simulink model "RL_GHV_open_smc"  (R2023b)
settings: Solver=VariableStepAuto  StartTime=0  StopTime=5  FixedStep=0.01  MaxStep=0.001  RelTol=1e-3
model workspace (MAT data in the model file):
  initPosLLA = [0; 0; 30000]
values from neighbouring files (symbols this model uses):
  Vm_0 = [speed_0; 0; 0]    [init_RL_GHV_open_evn_agent.m]
undefined symbols (not defined in the file or in its folder): e0_0, e1_0, e2_0, e3_0, GHV_cfg, LLA_init, pm_0, Speed_init
libraries: aerolib6dof2 x6, sharedutil x4, aerolibtransform2 x4, sharedtransform x4, simulink_extras x4, shared6dofsys x3, aerolibasang x3, aerolibatmos2 x1, matrix_library x1, aerolibgravity2 x1, rllib x1
settings Model: SimulationMode=accelerator  Creator=Admin  LastModifiedBy=Admin
settings SolverCC: AllowMultiTaskInputOutput=on  ZeroCrossControl=EnableAll  ZeroCrossAlgorithm=Adaptive  AutoInsertRateTranBlk=on
settings DebuggingCC: IgnoredZcDiagnostic=none

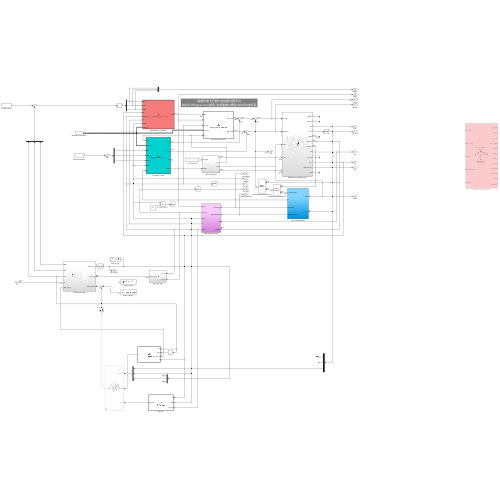
[thumbnail: Simulink's stored preview of the top-level diagram]
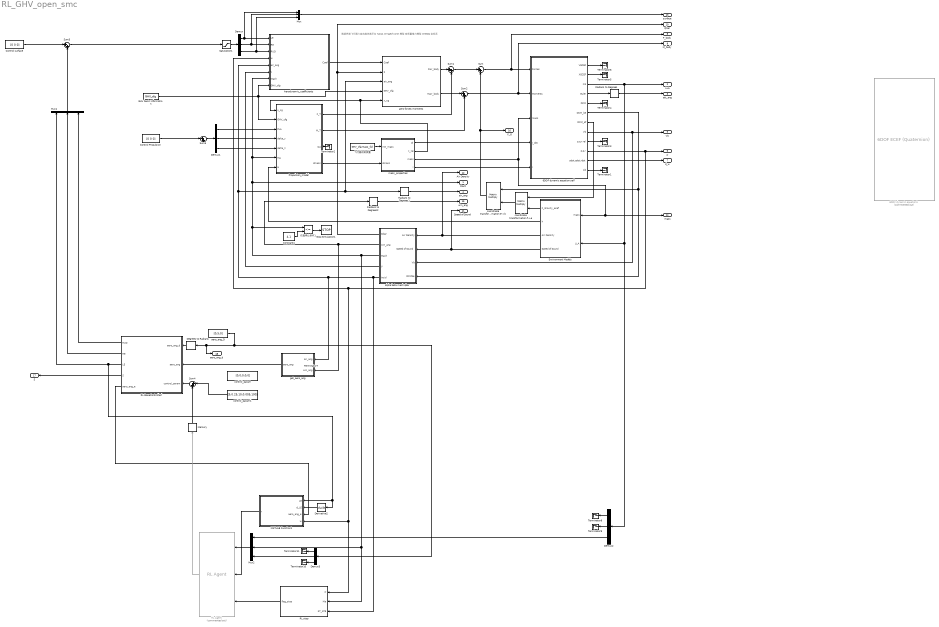
== system RL_GHV_open_smc ==
  note: 高超声速飞行器六自由度仿真平台
      | NASA Winged-cone模型 变质量推力模型 WGS84坐标系
  6DOF dynamic equation self : Subsystem
  6DOF dynamic equation1 : aerolib6dof2/6DOF ECEF (Quaternion)  Commented=on  units=Metric (MKS)  mtype=Custom Variable  xg_0=[0;0;20000]  Vm_0=[1475.347986769521;0;0]  eul_0=[0;0;0]  pm_0=[0;0;0]  mass_0=1.0  mass_e=0.5  mass_f=2.0  inertia=eye(3)  inertia_e=eye(3)  inertia_f=2*eye(3)  vre_flag=off  abi_flag=off  ptype=Custom  R=6378137  F=1/298.257223563  w_E=0  angle_in=Internal  LPM0=0  quat_statename=''  pm_statename=''  Vm_statename=''  posfixedframe_statename=''  posinertial_statename=''  LPM_statename=''  mass_statename=''
      settings: LibrarySourceBlock=|
      | aerolib6dof2/Custom Variable Mass 6DOF
      | ECEF (Quaternion)
  Aerodynamic_coefficients : MATLAB Function  TreatAsAtomicUnit=on
  Constant1 : Constant  Value=4.1
  Control Propulsion : Constant  Value=[0 0 0]
  Control surface : Constant  Value=[0 0 0]
  Degrees to Radians : simulink_extras/Transformations/Degrees to Radians
  Demux{,1..3} (4 alike) : Demux  Outputs=3
  Derivative2 : Derivative
  Environment Models : Subsystem
  GHV basic information : Constant  Value=GHV_cfg  VectorParams1D=off  OutDataTypeStr=Bus: slBus1
  MATLAB Function1 : MATLAB Function  TreatAsAtomicUnit=on
  Memory : Memory
  Mux : Mux  Inputs=3
  Mux1 : Mux  Inputs=3
  Mux2 : Mux  Inputs=3
  Propulsion_model : MATLAB Function  TreatAsAtomicUnit=on
  RL Agent : rllib/RL Agent  Commented=on  Agent=agent1_Trained  ExternalActionAsInput=off  ProvideLastAction=off  ProvideCumRwd=off  TreatAsDirectFeedthrough=on  UseStrictObservationDataTypes=off
  RL BaseControllerl : Subsystem
  RL stop : MATLAB Function  TreatAsAtomicUnit=on
  Radians to Degrees : simulink_extras/Transformations/Radians to Degrees
  Radians to Degrees1 : simulink_extras/Transformations/Radians to Degrees
  Radians to Degrees2 : simulink_extras/Transformations/Radians to Degrees
  Saturation1 : Saturate  UpperLimit=30  LowerLimit=-30
  Stop Simulation1 : Stop
  Sum{,1..5} (6 alike) : Sum  Inputs=|++
  Terminator{1..11} (11 alike) : Terminator
  aero forces moments : MATLAB Function  TreatAsAtomicUnit=on
  aero_ang_D : Constant  Value=[0;5;0]
  alpha beta mach qbar : Subsystem
  control_param : Constant  Value=[0;0;0;0;0]
  control_param1 : Constant  Value=[5;0.25;10;0.005;100]
  coordinate transformation e->b : Product  Multiplication=Matrix(*)
  coordinate transformation f->e : Product  Multiplication=Matrix(*)
  get_aero_ang : Subsystem
  mass_properties : Subsystem
  仿真停止条件1 : RelationalOperator  Operator=<=  OutDataTypeStr=boolean  RndMeth=Simplest  InputSameDT=off
  飞行器初始质量 : Constant  Value=GHV_cfg.mass_full
  Mach : Outport
  LLA : Outport  Port=2
  att_ang : Outport  Port=3
  air_ang : Outport  Port=4
  Vb : Outport  Port=5
  w : Outport  Port=6
  d_w : Outport  Port=7
  F_body : Outport  Port=8
  M_body : Outport  Port=9
  Qbar : Outport  Port=10
  Speed of Sound : Outport  Port=11
  Air Density : Outport  Port=12
  surface : Outport  Port=13
  mass : Outport  Port=14
  win_ang : Outport  Port=15
  F_G : Outport  Port=16
  S : Outport  Port=17
  aero_ang_d : Outport  Port=18
  wires:
  Control surface/1 -> Sum3/1
  coordinate transformation e->b/1 -> F_G/1, Sum/2
  Aerodynamic_coefficients/1(Coef) -> aero forces moments/1(Coef)
  mass_properties/2(x_cg) -> Propulsion_model/1(x_cg), aero forces moments/5(x_cg)
  coordinate transformation f->e/1 -> coordinate transformation e->b/2
  飞行器初始质量/1 -> mass_properties/1(init_mass)
  Radians to Degrees1/1 -> air_ang/1
  Propulsion_model/2(M_T) -> Sum2/2
  6DOF dynamic equation self/1(VECEF) -> Terminator6/1
  6DOF dynamic equation self/9(p,q,r rel) -> Terminator3/1
  mass_properties/3(mass) -> 6DOF dynamic equation self/3(mass), Environment Models/1(mass), mass/1
  Radians to Degrees2/1 -> win_ang/1
  Demux/1 -> Aerodynamic_coefficients/1(LE), Mux/1
  6DOF dynamic equation self/5(DCM) -> Terminator4/1
  Saturation1/1 -> Demux/1
  Demux1/2 -> Propulsion_model/4(delta_y)
  Control Propulsion/1 -> Sum5/1
  Propulsion_model/1(F_T) -> Sum1/2
  6DOF dynamic equation self/3(XG) -> LLA/1, Environment Models/2(LLA), Demux2/1
  Demux/2 -> Aerodynamic_coefficients/2(RE), Mux/2
  alpha beta mach qbar/5(Incid) -> aero forces moments/3(air_ang), Radians to Degrees1/1, Aerodynamic_coefficients/5(air_ang), get_aero_ang/1(air_ang), RL stop/3(air_ang)
  Sum2/1 -> 6DOF dynamic equation self/2(Moments), M_body/1
  Propulsion_model/4(dmass) -> mass_properties/2(dmass)
  Sum1/1 -> Sum/1
  Environment Models/3(Air Density) -> alpha beta mach qbar/1(Air Density), Air Density/1
  Environment Models/2(h) -> Propulsion_model/7(H)
  alpha beta mach qbar/1(Qbar) -> aero forces moments/2(q), Qbar/1
  aero forces moments/1(Fair_body) -> Sum1/1
  Radians to Degrees/1 -> att_ang/1
  6DOF dynamic equation self/6(DCM_be) -> alpha beta mach qbar/4(DCMbe), coordinate transformation e->b/1
  aero forces moments/2(Mair_body) -> Sum2/1
  Demux1/3 -> Propulsion_model/5(delta_z)
  6DOF dynamic equation self/10(p,q,r) -> w/1, RL stop/1(w), MATLAB Function1/4(w), Aerodynamic_coefficients/4(w)
  Mux/1 -> surface/1
  GHV basic information/1 -> Propulsion_model/2(GHV_cfg), aero forces moments/4(GHV_cfg), Aerodynamic_coefficients/8(GHV_cfg)
  Demux/3 -> Aerodynamic_coefficients/3(RUD), Mux/3
  alpha beta mach qbar/2(win_ang) -> Radians to Degrees2/1, get_aero_ang/2(win_ang)
  Sum3/1 -> Saturation1/1
  Propulsion_model/3(Isp) -> Terminator2/1
  Environment Models/1(F_Gravity_ecef) -> coordinate transformation f->e/2
  6DOF dynamic equation self/11(pdot,qdot,rdot) -> d_w/1
  Demux1/1 -> Propulsion_model/3(PLA)
  mass_properties/1(dI) -> 6DOF dynamic equation self/4(I_dot)
  6DOF dynamic equation self/7(DCM_ef) -> coordinate transformation f->e/1
  6DOF dynamic equation self/2(XECEF) -> Terminator5/1
  6DOF dynamic equation self/8(Vb) -> Vb/1, alpha beta mach qbar/3(Vb)
  alpha beta mach qbar/4(V) -> Aerodynamic_coefficients/6(v)
  Environment Models/4(Speed of Sound) -> alpha beta mach qbar/2(Speed of Sound), Speed of Sound/1
  6DOF dynamic equation self/12(Ab) -> Terminator1/1
  6DOF dynamic equation self/4(Euler) -> Radians to Degrees/1
  Sum/1 -> 6DOF dynamic equation self/1(Forces), F_body/1
  mass_properties/4(I) -> 6DOF dynamic equation self/5(I)
  Sum5/1 -> Demux1/1
  alpha beta mach qbar/3(Mach) -> 仿真停止条件1/1, Mach/1, Propulsion_model/6(Ma), Aerodynamic_coefficients/7(Mach), RL stop/2(Ma), Mux2/2
  Mux1/1 -> Sum3/2
  Constant1/1 -> 仿真停止条件1/2
  仿真停止条件1/1 -> Stop Simulation1/1
  get_aero_ang/1(aero_ang) -> RL BaseControllerl/2(aero_ang)
  aero_ang_D/1 -> Demux3/1, aero_ang_d/1, Degrees to Radians/1
  RL BaseControllerl/1(RUD) -> Mux1/3
  RL BaseControllerl/2(RE) -> Mux1/2
  RL BaseControllerl/3(LE) -> MATLAB Function1/1(LE), Derivative2/1, Mux1/1
  RL BaseControllerl/4(S) -> S/1
  Degrees to Radians/1 -> RL BaseControllerl/1(aero_ang_d)
  Sum4/1 -> RL BaseControllerl/3(control_param)
  RL stop/1(flag_stop) -> RL Agent/3
  RL BaseControllerl/5(aero_ang_e) -> MATLAB Function1/3(aero_ang_e)
  MATLAB Function1/1(r) -> RL Agent/2
  Mux2/1 -> RL Agent/1
  Demux2/1 -> Terminator8/1
  Demux2/2 -> Terminator9/1
  Demux2/3 -> Mux2/1
  RL Agent/1 -> Memory/1
  control_param1/1 -> Sum4/1
  Derivative2/1 -> MATLAB Function1/2(d_LE)
  Demux3/2 -> Mux2/3
  Demux3/3 -> Terminator10/1
  Demux3/1 -> Terminator11/1
  Memory/1 -> Sum4/2

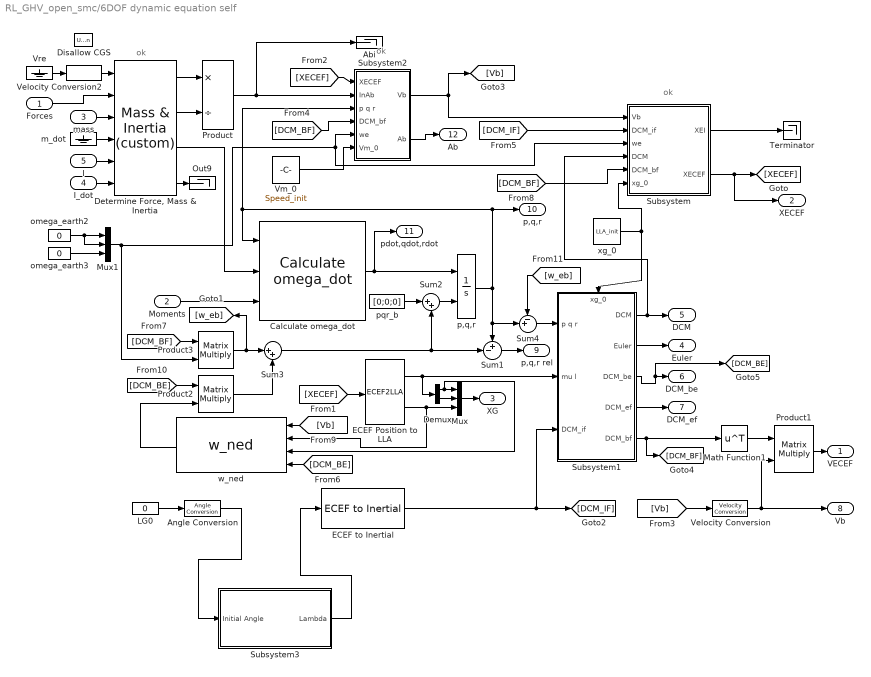
== system RL_GHV_open_smc/6DOF dynamic equation self ==
  note: ok
  note: ok
  note: ok
  Forces : Inport  OutDataTypeStr=double  Unit=N  PortDimensions=3
  Moments : Inport  Port=2  OutDataTypeStr=double  Unit=N*m  PortDimensions=3
  mass : Inport  Port=3  Unit=kg
  I_dot : Inport  Port=4  Unit=kg*m^2/s  PortDimensions=[3 3]
  I : Inport  Port=5  Unit=kg*m^2  PortDimensions=[3 3]
  Abi : Terminator
  Angle Conversion : aerolib6dof2/6DOF ECEF (Quaternion)/Angle Conversion  SystemSampleTime=-1  VariantActivationTime=update diagram  AllowFlexibleInterface=on  Latency=0  AutoFrameSizeCalculation=off
  Calculate omega_dot : shared6dofsys/Calculate omega_dot  aMode=aMode
  Demux : Demux  Outputs=2
  "Determine Force, Mass & Inertia" : shared6dofsys/Mass & Inertia (custom)  aMode=aMode
  Disallow CGS : UnitConfiguration  UnitSystemsStr=English,SI,SI (extended)  AllowAllUnitSystems=off
  ECEF Position to LLA : ECEF2LLA  ptype=Custom  R=6378137
  ECEF to Inertial : aerolib6dof2/6DOF ECEF (Quaternion)/ECEF to Inertial  SystemSampleTime=-1  VariantActivationTime=update diagram  AllowFlexibleInterface=on  Latency=0  AutoFrameSizeCalculation=off
  LG0 : Constant  Value=0  OutDataTypeStr=Inherit: Inherit via back propagation
  Math Function1 : Math  Operator=transpose  SignedPower=on
  Mux : Mux  Inputs=3
  Mux1 : Mux  Inputs=3
  Out9 : Terminator
  Product : Product  Inputs=*/  SaturateOnIntegerOverflow=on  OutDataTypeStr=Inherit: Same as first input
  Product1 : Product  Multiplication=Matrix(*)  RndMeth=Zero
  Product2 : Product  Multiplication=Matrix(*)  RndMeth=Zero
  Product3 : Product  Multiplication=Matrix(*)  RndMeth=Zero
  Subsystem : Subsystem
  Subsystem1 : Subsystem
      settings: PortSchema="{\"entries\":[{\"content\":{\"sides\":[{\"content\":{\"connectorIds\":[\"In1\",\"In2\",\"In3\"]},\"type\":\"ConnectorPlacement.EquallySpacedRectSide\",\"uuid\":\"53d15541-d89e-48eb-840a-d42af95f99e9\"},{\"content\":{\"connectorIds\":[\"Out1\",\"Out2\",\"Out3\",\"Out4\",\"Out5\"],\"side\":\"RIGHT\"},\"type\":\"ConnectorPlacement.EquallySpacedRectSide\",\"uuid\":\"e27a62cc-5eeb-4e70-bfca-60e5b3304488\"},{\"content\":{\"connectorIds\":[\"In4\"],\"side\":\"TOP\"},\"type\":\"ConnectorPlacement.EquallySpacedRectSide\",\"uuid\":\"1e26f7fc-1378-4117-9ebe-39004b309270\"}]},\"type\":\"ConnectorPlacement.EquallySpacedConnector\",\"uuid\":\"3afc0320-367d-4357-b7bd-bc22d5ec0517\"}],\"packageUris\":[\"http://schema.mathworks.com/mf0/Connector/R2020b\"],\"version\":\"1.0\"}"
  Subsystem2 : Subsystem
  Subsystem3 : Subsystem
  Sum1 : Sum  Inputs=+-|
  Sum2 : Sum  Inputs=|++
  Sum3 : Sum  Inputs=|++
  Sum4 : Sum  Inputs=-+|
  Terminator : Terminator
  Velocity Conversion : aerolib6dof2/6DOF ECEF (Quaternion)/Velocity Conversion  SystemSampleTime=-1  VariantActivationTime=update diagram  AllowFlexibleInterface=on  Latency=0  AutoFrameSizeCalculation=off
  Velocity Conversion2 : aerolib6dof2/6DOF ECEF (Quaternion)/Velocity Conversion2  SystemSampleTime=-1  VariantActivationTime=update diagram  AllowFlexibleInterface=on  Latency=0  AutoFrameSizeCalculation=off
  Vm_0 : Constant  Value=Speed_init
  Vre : Ground
  m_dot : Ground
  omega_earth2 : Constant  Value=0
  omega_earth3 : Constant  Value=0
  "p,q,r " : Integrator  InitialConditionSource=external  InitialCondition=pm_0
  pqr_b : Constant  Value=[0;0;0]
  w_ned : aerolib6dof2/6DOF ECEF (Quaternion)/w_ned  SystemSampleTime=-1  VariantActivationTime=update diagram  AllowFlexibleInterface=on  Latency=0  AutoFrameSizeCalculation=off
      link override M+h/f1: Value=6378137
      link override N+h/f4: Value=6378137
      link override e2/Constant: Value=1/298.257223563
  xg_0 : Constant  Value=LLA_init
  VECEF : Outport  OutDataTypeStr=double  Unit=m/s  VectorParamsAs1DForOutWhenUnconnected=off
  XECEF : Outport  Port=2  OutDataTypeStr=double  Unit=m  VectorParamsAs1DForOutWhenUnconnected=off
  XG : Outport  Port=3  OutDataTypeStr=double  VectorParamsAs1DForOutWhenUnconnected=off
  Euler : Outport  Port=4  OutDataTypeStr=double  Unit=rad  VectorParamsAs1DForOutWhenUnconnected=off
  DCM : Outport  Port=5  OutDataTypeStr=double  Unit=1  VectorParamsAs1DForOutWhenUnconnected=off
  DCM_be : Outport  Port=6  OutDataTypeStr=double  Unit=1  VectorParamsAs1DForOutWhenUnconnected=off
  DCM_ef : Outport  Port=7  OutDataTypeStr=double  Unit=1  VectorParamsAs1DForOutWhenUnconnected=off
  Vb : Outport  Port=8  OutDataTypeStr=double  Unit=m/s  VectorParamsAs1DForOutWhenUnconnected=off
  p,q,r rel : Outport  Port=9  OutDataTypeStr=double  Unit=rad/s  VectorParamsAs1DForOutWhenUnconnected=off
  p,q,r : Outport  Port=10  OutDataTypeStr=double  Unit=rad/s  VectorParamsAs1DForOutWhenUnconnected=off
  pdot,qdot,rdot : Outport  Port=11  OutDataTypeStr=double  Unit=rad/s^2  VectorParamsAs1DForOutWhenUnconnected=off
  Ab : Outport  Port=12  OutDataTypeStr=double  Unit=m/s^2  VectorParamsAs1DForOutWhenUnconnected=off
  wires:
  Subsystem/2(XECEF) -> [XECEF], XECEF/1
  Subsystem1/5(DCM_bf) -> Math Function1/1, [DCM_BF]
  Product3/1 -> [w_eb], Sum3/1
  Subsystem1/1(DCM) -> DCM/1, Subsystem/4(DCM)
  Subsystem1/4(DCM_ef) -> DCM_ef/1
  [DCM_IF] -> Subsystem/2(DCM_if)
  Product1/1 -> VECEF/1
  [Vb] -> Velocity Conversion/1
  Mux/1 -> XG/1
  [DCM_BE] -> Product2/1
  Forces/1 -> "Determine Force, Mass & Inertia"/2
  Math Function1/1 -> Product1/1
  [DCM_BF] -> Subsystem/5(DCM_bf)
  Product/1 -> Subsystem2/2(InAb), Abi/1
  omega_earth2/1 -> Mux1/1, Mux1/2
  Angle Conversion/1 -> Subsystem3/1(Initial Angle)
  ECEF Position to LLA/2 -> Mux/3, w_ned/2
  ECEF Position to LLA/1 -> Subsystem1/2(mu l), Demux/1
  Subsystem1/2(Euler) -> Euler/1
  Sum3/1 -> Sum2/2, Sum1/2
  [XECEF] -> Subsystem2/1(XECEF)
  omega_earth3/1 -> Mux1/3
  w_ned/1 -> Product2/2
  [Vb] -> w_ned/1
  Sum4/1 -> Subsystem1/1(p q r)
  [XECEF] -> ECEF Position to LLA/1
  Velocity Conversion/1 -> Product1/2, Vb/1
  ECEF to Inertial/1 -> Subsystem1/3(DCM_if), [DCM_IF]
  Sum1/1 -> p,q,r rel/1
  I/1 -> "Determine Force, Mass & Inertia"/5
  "Determine Force, Mass & Inertia"/1 -> Product/1
  m_dot/1 -> "Determine Force, Mass & Inertia"/4
  pqr_b/1 -> Sum2/1
  Product2/1 -> Sum3/2
  I_dot/1 -> "Determine Force, Mass & Inertia"/6
  "Determine Force, Mass & Inertia"/2 -> Product/2
  [DCM_BF] -> Product3/1
  [DCM_BE] -> w_ned/4
  [w_eb] -> Sum4/1
  "Determine Force, Mass & Inertia"/4 -> Out9/1
  Vre/1 -> Velocity Conversion2/1
  Subsystem/1(XEI) -> Terminator/1
  Demux/1 -> w_ned/3, Mux/1
  Subsystem1/3(DCM_be) -> DCM_be/1, [DCM_BE]
  "Determine Force, Mass & Inertia"/3 -> Calculate omega_dot/2
  Calculate omega_dot/1 -> pdot,qdot,rdot/1, "p,q,r "/1
  Subsystem3/1(Lambda) -> ECEF to Inertial/1
  Moments/1 -> Calculate omega_dot/3
  [DCM_BF] -> Subsystem2/4(DCM_bf)
  Sum2/1 -> "p,q,r "/2
  Demux/2 -> Mux/2
  LG0/1 -> Angle Conversion/1
  Subsystem2/2(Ab) -> Ab/1
  mass/1 -> "Determine Force, Mass & Inertia"/3
  Velocity Conversion2/1 -> "Determine Force, Mass & Inertia"/1
  Subsystem2/1(Vb) -> [Vb], Subsystem/1(Vb)
  Mux1/1 -> Subsystem2/5(we), Subsystem/3(we), Product3/2
  "p,q,r "/1 -> Subsystem2/3(p q r), Calculate omega_dot/1, p,q,r/1, Sum4/2, Sum1/1
  Vm_0/1 -> Subsystem2/6(Vm_0)
  xg_0/1 -> Subsystem/6(xg_0), Subsystem1/4(xg_0)

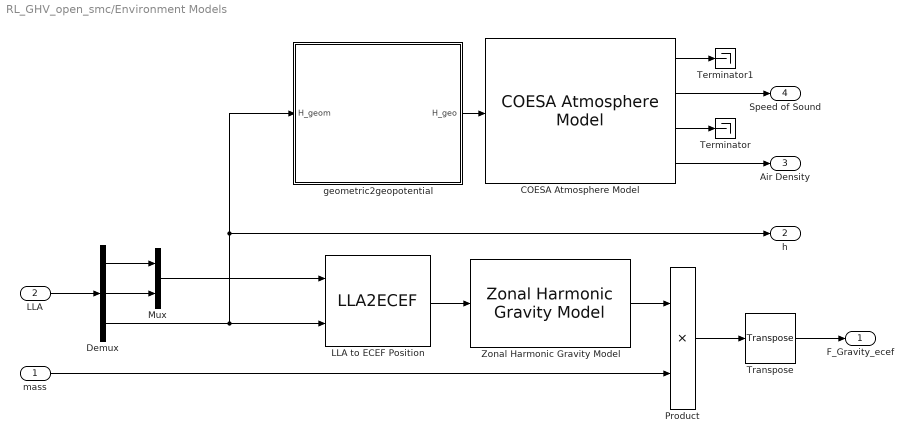
== system RL_GHV_open_smc/Environment Models ==
  mass : Inport
  LLA : Inport  Port=2
  COESA Atmosphere Model : aerolibatmos2/COESA Atmosphere Model  units=Metric (MKS)  spec=1976 COESA-extended U.S. Standard Atmosphere  model=Profile  profile_var=High temperature  profile_percent=1%  profile_alt=5 km (16404 ft)  envelope_var=High temperature  envelope_percent=1%  action=Warning
  Demux : Demux  Outputs=3
  LLA to ECEF Position : LLA2ECEF
  Mux : Mux  Inputs=2
  Product : Product
  Terminator : Terminator
  Terminator1 : Terminator
  Transpose : matrix_library/Transpose
  Zonal Harmonic Gravity Model : aerolibgravity2/Zonal Harmonic Gravity Model  units=Metric (MKS)  degree=2  action=Warning  ptype=Earth  R=6378136.3  GM=398600441500000  jvalue=[1.0826269e-03 -2.5323000e-06 -1.6204000e-06]
  geometric2geopotential : MATLAB Function  TreatAsAtomicUnit=on
  F_Gravity_ecef : Outport
  h : Outport  Port=2
  Air Density : Outport  Port=3
  Speed of Sound : Outport  Port=4
  wires:
  COESA Atmosphere Model/1 -> Terminator1/1
  COESA Atmosphere Model/2 -> Speed of Sound/1
  COESA Atmosphere Model/3 -> Terminator/1
  COESA Atmosphere Model/4 -> Air Density/1
  LLA to ECEF Position/1 -> Zonal Harmonic Gravity Model/1
  Mux/1 -> LLA to ECEF Position/1
  Demux/3 -> h/1, geometric2geopotential/1(H_geom), LLA to ECEF Position/2
  Demux/1 -> Mux/1
  Demux/2 -> Mux/2
  LLA/1 -> Demux/1
  mass/1 -> Product/2
  Zonal Harmonic Gravity Model/1 -> Product/1
  Product/1 -> Transpose/1
  Transpose/1 -> F_Gravity_ecef/1
  geometric2geopotential/1(H_geo) -> COESA Atmosphere Model/1

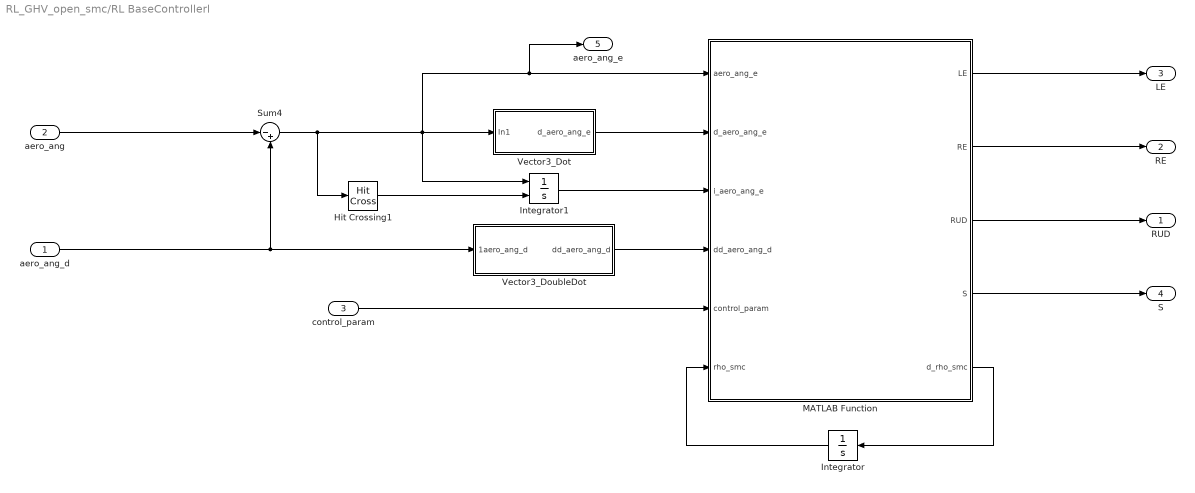
== system RL_GHV_open_smc/RL BaseControllerl ==
  aero_ang_d : Inport
  aero_ang : Inport  Port=2
  control_param : Inport  Port=3
  Hit Crossing1 : HitCross
  Integrator : Integrator  InitialCondition=[0;10;0]
  Integrator1 : Integrator  ExternalReset=either
  MATLAB Function : MATLAB Function  TreatAsAtomicUnit=on
  Sum4 : Sum  Inputs=|-+
  Vector3_Dot : Subsystem
  Vector3_DoubleDot : Subsystem
  RUD : Outport
  RE : Outport  Port=2
  LE : Outport  Port=3
  S : Outport  Port=4
  aero_ang_e : Outport  Port=5
  wires:
  control_param/1 -> MATLAB Function/5(control_param)
  Vector3_Dot/1(d_aero_ang_e) -> MATLAB Function/2(d_aero_ang_e)
  Vector3_DoubleDot/1(dd_aero_ang_d) -> MATLAB Function/4(dd_aero_ang_d)
  MATLAB Function/5(d_rho_smc) -> Integrator/1
  MATLAB Function/2(RE) -> RE/1
  aero_ang_d/1 -> Sum4/2, Vector3_DoubleDot/1(1aero_ang_d)
  MATLAB Function/1(LE) -> LE/1
  Integrator1/1 -> MATLAB Function/3(i_aero_ang_e)
  MATLAB Function/3(RUD) -> RUD/1
  MATLAB Function/4(S) -> S/1
  Integrator/1 -> MATLAB Function/6(rho_smc)
  Sum4/1 -> Hit Crossing1/1, aero_ang_e/1, MATLAB Function/1(aero_ang_e), Integrator1/1, Vector3_Dot/1(In1)
  aero_ang/1 -> Sum4/1
  Hit Crossing1/1 -> Integrator1/2

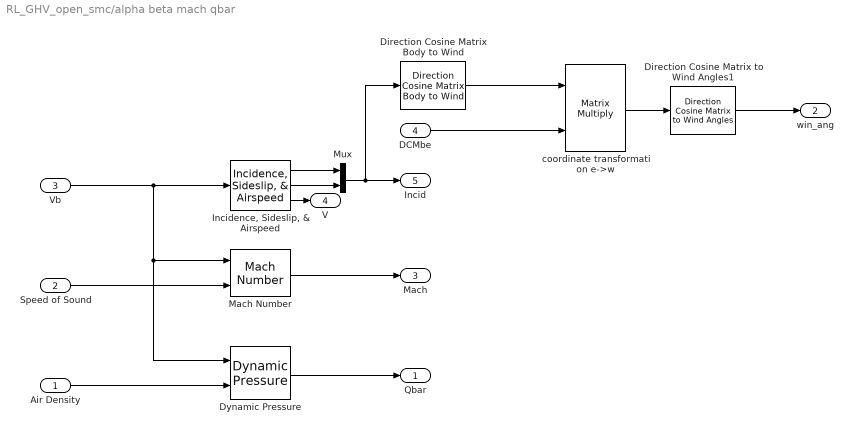
== system RL_GHV_open_smc/alpha beta mach qbar ==
  Air Density : Inport
  Speed of Sound : Inport  Port=2
  Vb : Inport  Port=3
  DCMbe : Inport  Port=4
  Direction Cosine Matrix Body to Wind : aerolibtransform2/Direction Cosine Matrix Body to Wind
  Direction Cosine Matrix to Wind Angles1 : aerolibtransform2/Direction Cosine Matrix to Wind Angles  action=None  tolerance=eps(2)
  Dynamic Pressure : aerolibasang/Dynamic Pressure
  "Incidence, Sideslip, & Airspeed" : aerolibasang/Incidence, Sideslip, & Airspeed
  Mach Number : aerolibasang/Mach Number
  Mux : Mux  Inputs=2
  coordinate transformation e->w : Product  Multiplication=Matrix(*)
  Qbar : Outport
  win_ang : Outport  Port=2
  Mach : Outport  Port=3
  V : Outport  Port=4
  Incid : Outport  Port=5
  wires:
  Speed of Sound/1 -> Mach Number/2
  Mach Number/1 -> Mach/1
  "Incidence, Sideslip, & Airspeed"/2 -> Mux/2
  Vb/1 -> Dynamic Pressure/1, Mach Number/1, "Incidence, Sideslip, & Airspeed"/1
  Dynamic Pressure/1 -> Qbar/1
  Mux/1 -> Direction Cosine Matrix Body to Wind/1, Incid/1
  "Incidence, Sideslip, & Airspeed"/1 -> Mux/1
  Air Density/1 -> Dynamic Pressure/2
  "Incidence, Sideslip, & Airspeed"/3 -> V/1
  DCMbe/1 -> coordinate transformation e->w/2
  Direction Cosine Matrix Body to Wind/1 -> coordinate transformation e->w/1
  coordinate transformation e->w/1 -> Direction Cosine Matrix to Wind Angles1/1
  Direction Cosine Matrix to Wind Angles1/1 -> win_ang/1

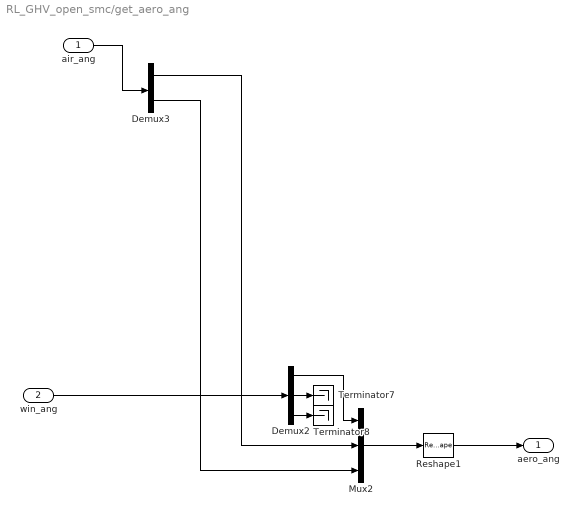
== system RL_GHV_open_smc/get_aero_ang ==
  air_ang : Inport
  win_ang : Inport  Port=2
  Demux2 : Demux  Outputs=3
  Demux3 : Demux  Outputs=2
  Mux2 : Mux  Inputs=3
  Reshape1 : Reshape  OutputDimensionality=Column vector (2-D)
  Terminator7 : Terminator
  Terminator8 : Terminator
  aero_ang : Outport
  wires:
  Mux2/1 -> Reshape1/1
  Demux2/2 -> Terminator7/1
  Reshape1/1 -> aero_ang/1
  air_ang/1 -> Demux3/1
  Demux3/1 -> Mux2/2
  win_ang/1 -> Demux2/1
  Demux2/3 -> Terminator8/1
  Demux3/2 -> Mux2/3
  Demux2/1 -> Mux2/1

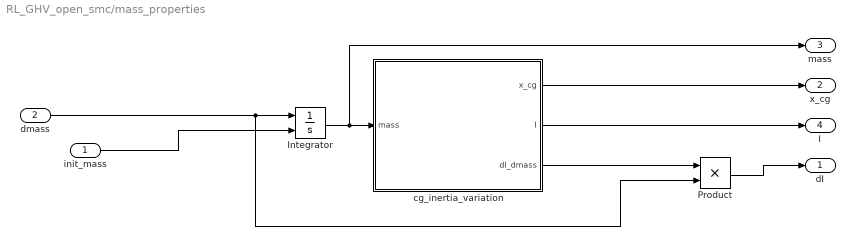
== system RL_GHV_open_smc/mass_properties ==
  init_mass : Inport
  dmass : Inport  Port=2
  Integrator : Integrator  InitialConditionSource=external
  Product : Product
  cg_inertia_variation : MATLAB Function  TreatAsAtomicUnit=on
  dI : Outport
  x_cg : Outport  Port=2
  mass : Outport  Port=3
  I : Outport  Port=4
  wires:
  Integrator/1 -> mass/1, cg_inertia_variation/1(mass)
  init_mass/1 -> Integrator/2
  cg_inertia_variation/3(dI_dmass) -> Product/1
  dmass/1 -> Product/2, Integrator/1
  cg_inertia_variation/2(I) -> I/1
  cg_inertia_variation/1(x_cg) -> x_cg/1
  Product/1 -> dI/1

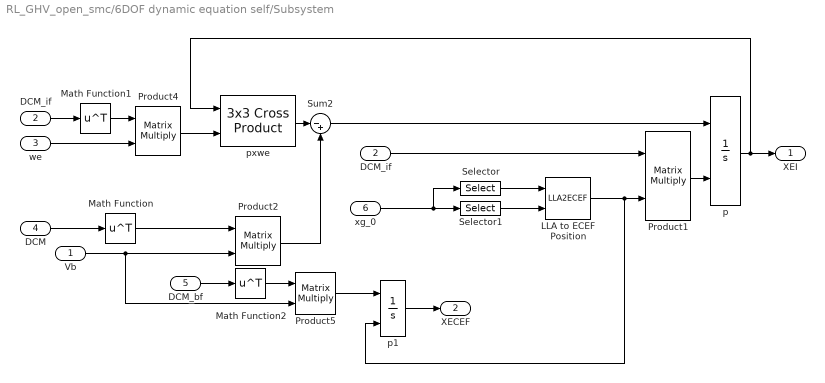
== system RL_GHV_open_smc/6DOF dynamic equation self/Subsystem ==
  Vb : Inport
  DCM_if : Inport  Port=2
  we : Inport  Port=3
  DCM : Inport  Port=4
  DCM_bf : Inport  Port=5
  xg_0 : Inport  Port=6
  "DCM_if " : InportShadow  Port=2
  LLA to ECEF Position : LLA2ECEF  ptype=Custom  R=6378137
  Math Function : Math  Operator=transpose  SignedPower=on
  Math Function1 : Math  Operator=transpose  SignedPower=on
  Math Function2 : Math  Operator=transpose  SignedPower=on
  Product{1..2,4..5} (4 alike) : Product  Multiplication=Matrix(*)  RndMeth=Zero
  Selector : Selector  InputPortWidth=3  IndexOptions=Index vector (dialog)  Indices=[1 2]  OutputSizes=1
  Selector1 : Selector  InputPortWidth=3  IndexOptions=Index vector (dialog)  Indices=[3]  OutputSizes=1
  Sum2 : Sum  Inputs=|-+  SaturateOnIntegerOverflow=on
  p : Integrator  InitialConditionSource=external
  p1 : Integrator  InitialConditionSource=external
  pxwe : sharedutil/3x3 Cross Product  aMode=aMode
  XEI : Outport  VectorParamsAs1DForOutWhenUnconnected=off
  XECEF : Outport  Port=2  VectorParamsAs1DForOutWhenUnconnected=off
  wires:
  Math Function1/1 -> Product4/1
  DCM_bf/1 -> Math Function2/1
  Product2/1 -> Sum2/2
  Selector/1 -> LLA to ECEF Position/1
  xg_0/1 -> Selector/1, Selector1/1
  Math Function2/1 -> Product5/1
  Product4/1 -> pxwe/2
  p/1 -> pxwe/1, XEI/1
  p1/1 -> XECEF/1
  we/1 -> Product4/2
  "DCM_if "/1 -> Math Function1/1
  pxwe/1 -> Sum2/1
  DCM_if/1 -> Product1/1
  LLA to ECEF Position/1 -> p1/2, Product1/2
  DCM/1 -> Math Function/1
  Selector1/1 -> LLA to ECEF Position/2
  Vb/1 -> Product5/2, Product2/2
  Math Function/1 -> Product2/1
  Product5/1 -> p1/1
  Sum2/1 -> p/1
  Product1/1 -> p/2

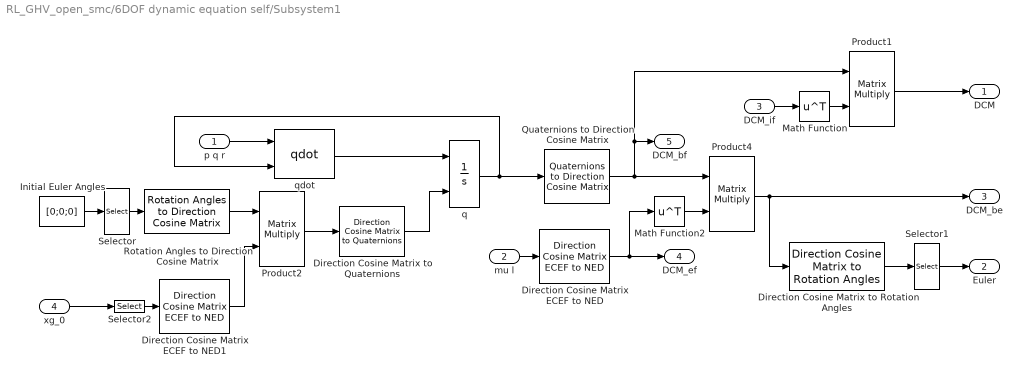
== system RL_GHV_open_smc/6DOF dynamic equation self/Subsystem1 ==
  p q r : Inport
  mu l : Inport  Port=2
  DCM_if : Inport  Port=3  PortDimensions=[3 3]
  xg_0 : Inport  Port=4
  Direction Cosine Matrix ECEF to NED : aerolibtransform2/Direction Cosine Matrix ECEF to NED
  Direction Cosine Matrix ECEF to NED1 : aerolibtransform2/Direction Cosine Matrix ECEF to NED
  Direction Cosine Matrix to Rotation Angles : sharedtransform/Direction Cosine Matrix to Rotation Angles  rotationOrder=ZYX  aMode=aMode  action=None  tolerance=eps(2)
  Direction Cosine Matrix to Quaternions : sharedtransform/Direction Cosine Matrix  to Quaternions  aMode=0  action=None  tolerance=eps(2)
  Initial Euler Angles : Constant  Value=[0;0;0]
  Math Function : Math  Operator=transpose  SignedPower=on
  Math Function2 : Math  Operator=transpose  SignedPower=on
  Product1 : Product  Multiplication=Matrix(*)  RndMeth=Zero
  Product2 : Product  Multiplication=Matrix(*)  RndMeth=Zero
  Product4 : Product  Multiplication=Matrix(*)  RndMeth=Zero
  Quaternions to Direction Cosine Matrix : sharedtransform/Quaternions to  Direction Cosine Matrix  aMode=aMode
  Rotation Angles to Direction Cosine Matrix : sharedtransform/Rotation Angles to Direction Cosine Matrix  rotationOrder=ZYX  aMode=aMode
  Selector : Selector  InputPortWidth=3  IndexOptions=Index vector (dialog)  Indices=[3 2 1]  OutputSizes=1
  Selector1 : Selector  InputPortWidth=3  IndexOptions=Index vector (dialog)  Indices=[3 2 1]  OutputSizes=1
  Selector2 : Selector  InputPortWidth=3  IndexOptions=Index vector (dialog)  Indices=[1 2]  OutputSizes=1
  q : Integrator  InitialConditionSource=external  InitialCondition=[e0_0 e1_0 e2_0 e3_0]
  qdot : shared6dofsys/qdot  aMode=aMode
  DCM : Outport  VectorParamsAs1DForOutWhenUnconnected=off
  Euler : Outport  Port=2  VectorParamsAs1DForOutWhenUnconnected=off
  DCM_be : Outport  Port=3  VectorParamsAs1DForOutWhenUnconnected=off
  DCM_ef : Outport  Port=4  VectorParamsAs1DForOutWhenUnconnected=off
  DCM_bf : Outport  Port=5  VectorParamsAs1DForOutWhenUnconnected=off
  wires:
  q/1 -> Quaternions to Direction Cosine Matrix/1, qdot/2
  Selector1/1 -> Euler/1
  Direction Cosine Matrix ECEF to NED/1 -> Math Function2/1, DCM_ef/1
  Math Function2/1 -> Product4/2
  Product2/1 -> Direction Cosine Matrix to Quaternions/1
  qdot/1 -> q/1
  mu l/1 -> Direction Cosine Matrix ECEF to NED/1
  Quaternions to Direction Cosine Matrix/1 -> Product4/1, DCM_bf/1, Product1/1
  Math Function/1 -> Product1/2
  Direction Cosine Matrix to Quaternions/1 -> q/2
  p q r/1 -> qdot/1
  Product4/1 -> DCM_be/1, Direction Cosine Matrix to Rotation Angles/1
  DCM_if/1 -> Math Function/1
  Direction Cosine Matrix to Rotation Angles/1 -> Selector1/1
  Product1/1 -> DCM/1
  Rotation Angles to Direction Cosine Matrix/1 -> Product2/1
  Selector2/1 -> Direction Cosine Matrix ECEF to NED1/1
  xg_0/1 -> Selector2/1
  Selector/1 -> Rotation Angles to Direction Cosine Matrix/1
  Direction Cosine Matrix ECEF to NED1/1 -> Product2/2
  Initial Euler Angles/1 -> Selector/1

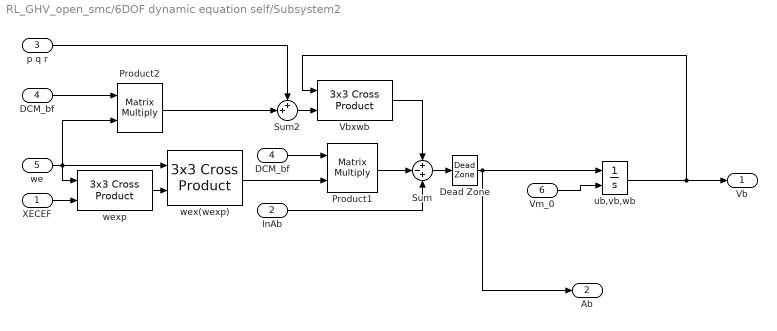
== system RL_GHV_open_smc/6DOF dynamic equation self/Subsystem2 ==
  XECEF : Inport
  InAb : Inport  Port=2
  p q r : Inport  Port=3
  DCM_bf : Inport  Port=4
  we : Inport  Port=5
  Vm_0 : Inport  Port=6
  "DCM_bf " : InportShadow  Port=4
  Dead Zone : DeadZone  LowerValue=-eps  UpperValue=eps
  Product1 : Product  Multiplication=Matrix(*)  RndMeth=Zero
  Product2 : Product  Multiplication=Matrix(*)  RndMeth=Zero
  Sum : Sum  Inputs=+-+  SaturateOnIntegerOverflow=on
  Sum2 : Sum  Inputs=++|  SaturateOnIntegerOverflow=on
  Vbxwb : sharedutil/3x3 Cross Product  aMode=aMode
  ub,vb,wb : Integrator  InitialConditionSource=external  InitialCondition=Vm_0
  wex(wexp) : sharedutil/3x3 Cross Product  aMode=aMode
  wexp : sharedutil/3x3 Cross Product  aMode=aMode
  Vb : Outport  VectorParamsAs1DForOutWhenUnconnected=off
  Ab : Outport  Port=2  VectorParamsAs1DForOutWhenUnconnected=off
  wires:
  ub,vb,wb/1 -> Vbxwb/1, Vb/1
  DCM_bf/1 -> Product1/1
  we/1 -> Product2/2, wexp/1, wex(wexp)/1
  Vbxwb/1 -> Sum/1
  XECEF/1 -> wexp/2
  wex(wexp)/1 -> Product1/2
  wexp/1 -> wex(wexp)/2
  Sum/1 -> Dead Zone/1
  Product2/1 -> Sum2/2
  "DCM_bf "/1 -> Product2/1
  InAb/1 -> Sum/3
  Dead Zone/1 -> Ab/1, ub,vb,wb/1
  p q r/1 -> Sum2/1
  Sum2/1 -> Vbxwb/2
  Product1/1 -> Sum/2
  Vm_0/1 -> ub,vb,wb/2

== system RL_GHV_open_smc/6DOF dynamic equation self/Subsystem3 ==
  Initial Angle : Inport  Unit=rad
  Constant1 : Constant  Value=0
  Integrator : Integrator
  Sum : Sum  Inputs=|++
  Lambda : Outport  VectorParamsAs1DForOutWhenUnconnected=off
  wires:
  Integrator/1 -> Sum/2
  Sum/1 -> Lambda/1
  Constant1/1 -> Integrator/1  "we"
  Initial Angle/1 -> Sum/1

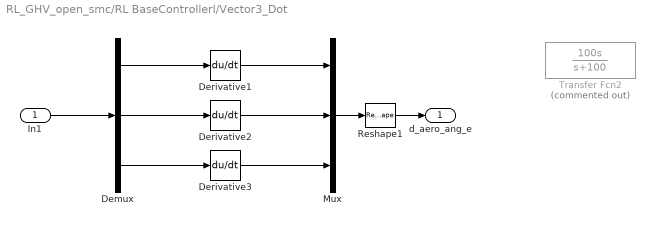
== system RL_GHV_open_smc/RL BaseControllerl/Vector3_Dot ==
  In1 : Inport
  Demux : Demux  Outputs=3
  Derivative1 : Derivative
  Derivative2 : Derivative
  Derivative3 : Derivative
  Mux : Mux  Inputs=3
  Reshape1 : Reshape  OutputDimensionality=Column vector (2-D)
  Transfer Fcn2 : TransferFcn  Commented=on  Numerator=[100 0]  Denominator=[1 100]
  d_aero_ang_e : Outport
  wires:
  In1/1 -> Demux/1
  Demux/2 -> Derivative2/1
  Demux/1 -> Derivative1/1
  Demux/3 -> Derivative3/1
  Mux/1 -> Reshape1/1
  Reshape1/1 -> d_aero_ang_e/1
  Derivative1/1 -> Mux/1
  Derivative2/1 -> Mux/2
  Derivative3/1 -> Mux/3

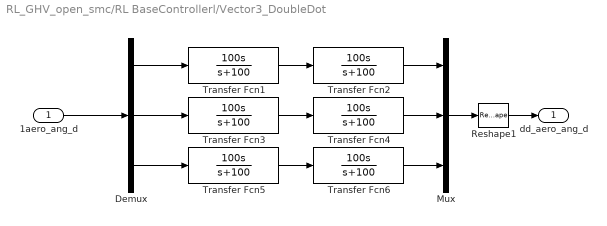
== system RL_GHV_open_smc/RL BaseControllerl/Vector3_DoubleDot ==
  1aero_ang_d : Inport
  Demux : Demux  Outputs=3
  Mux : Mux  Inputs=3
  Reshape1 : Reshape  OutputDimensionality=Column vector (2-D)
  Transfer Fcn{1..6} (6 alike) : TransferFcn  Numerator=[100 0]  Denominator=[1 100]
  dd_aero_ang_d : Outport
  wires:
  Transfer Fcn1/1 -> Transfer Fcn2/1
  1aero_ang_d/1 -> Demux/1
  Transfer Fcn3/1 -> Transfer Fcn4/1
  Transfer Fcn5/1 -> Transfer Fcn6/1
  Demux/2 -> Transfer Fcn3/1
  Demux/1 -> Transfer Fcn1/1
  Demux/3 -> Transfer Fcn5/1
  Transfer Fcn4/1 -> Mux/2
  Transfer Fcn6/1 -> Mux/3
  Transfer Fcn2/1 -> Mux/1
  Mux/1 -> Reshape1/1
  Reshape1/1 -> dd_aero_ang_d/1

== matlab function RL_GHV_open_smc/MATLAB Function1 ==
  data: LE input; d_LE input; aero_ang_e input; r output; w input
function r = S_reward(LE, d_LE, aero_ang_e, w)

   r = reward(aero_ang_e, w, LE, d_LE);

end

== matlab function RL_GHV_open_smc/Propulsion_model ==
  data: F_T output; M_T output; x_cg input; GHV_cfg input; PLA input; delta_y input; delta_z input; Ma input; H input; Isp output; dmass output
function [F_T,M_T, Isp,  dmass] = S_Propulsion_model(x_cg, GHV_cfg, PLA, delta_y, delta_z, Ma, H)
    F_T = zeros(3, 1); %#ok<PREALL>
    M_T = zeros(3, 1); %#ok<PREALL>
   [F_T, M_T, Isp, dmass] = Propulsion_model(PLA, H, Ma, delta_y, delta_z, GHV_cfg, x_cg);

end

== matlab function RL_GHV_open_smc/Aerodynamic_coefficients ==
  data: LE input; Coef output; RE input; RUD input; w input; air_ang input; v input; Mach input; GHV_cfg input
function Coef = S_Aerodynamic_coefficients(LE, RE, RUD, w, air_ang,v, Mach, GHV_cfg)
    Coef = zeros(6, 1);
    Coef = Aerodynamic_coefficients(LE, RE, RUD, air_ang, v, w, Mach, GHV_cfg);

end

== matlab function RL_GHV_open_smc/aero forces moments ==
  data: Coef input; q input; air_ang input; GHV_cfg input; x_cg input; Fair_body output; Mair_body output
function [Fair_body, Mair_body] = S_aero_forces_moments(Coef, q, air_ang, GHV_cfg, x_cg)

    Fair_body = zeros(3, 1); %#ok<PREALL>
    Mair_body = zeros(3, 1); %#ok<PREALL>
    [Fair_body, Mair_body] = aero_forces_moments(Coef, q, GHV_cfg, x_cg, air_ang);

end

== matlab function RL_GHV_open_smc/Environment Models/geometric2geopotential ==
  data: H_geom input; H_geo output
function H_geo = S_geometric2geopotential(H_geom)

    H_geo = geometric2geopotential(H_geom);

end

== matlab function RL_GHV_open_smc/RL BaseControllerl/MATLAB Function ==
  data: aero_ang_e input; d_aero_ang_e input; i_aero_ang_e input; dd_aero_ang_d input; LE output; control_param input; rho_smc input; RE output; RUD output; S output; d_rho_smc output
function [LE, RE, RUD, S, d_rho_smc] = S_RL_BaseController(aero_ang_e, d_aero_ang_e, i_aero_ang_e, dd_aero_ang_d, control_param, rho_smc)

 [LE, RE, RUD, d_rho_smc, S] = RL_BaseController(dd_aero_ang_d, aero_ang_e, d_aero_ang_e, i_aero_ang_e, rho_smc, control_param);

end

== matlab function RL_GHV_open_smc/RL stop ==
  data: w input; Ma input; air_ang input; flag_stop output
function flag_stop = S_RL_stop(w, Ma, air_ang)

 flag_stop = RL_stop(Ma, w, air_ang);

end

== matlab function RL_GHV_open_smc/mass_properties/cg_inertia_variation ==
  data: mass input; x_cg output; I output; dI_dmass output
function [x_cg, I, dI_dmass] = S_cg_inertia_variation(mass)

     [x_cg, I, dI_dmass] = cg_inertia_variation(mass);
     
end
